simulink model "lab6b"  (R2013b)
settings: Solver=ode3  StartTime=0.0  StopTime=10  FixedStep=0.002  RelTol=1e-3
undefined symbols (not defined in the file or in its folder): HIL
libraries: quarc_library x3
settings Model: SimulationMode=external  ExtModeTrigDuration=1000000  Creator=ee128-aat  LastModifiedBy=ee128-aat
settings SolverCC: PositivePriorityOrder=on
settings DataIOCC: LimitDataPoints=off
settings RTWCC: SystemTargetFile=quarc_win64.tlc  TemplateMakefile=quarc_default_tmf  Description=QUARC Win64 Target  ProcessScript=quarc_win64_make_rtw_hook
settings STFCustomTargetCC: TargetPreCompLibLocation=C:\PROGRA~3\QUARC\lib\2013b\win64\release  GeneratePreprocessorConditionals=Disable all  CombineOutputUpdateFcns=on  GRTInterface=off  SystemTargetFile=quarc_win64.tlc
settings GRTTargetCC: TargetPreCompLibLocation=C:\PROGRA~3\QUARC\lib\2013b\win64\release  ParMdlRefBuildCompliant=off  CompOptLevelCompliant=off  ConcurrentExecutionCompliant=off  MatFileLogging=off  ExtMode=on  ExtModeMexFile=quarc_comm

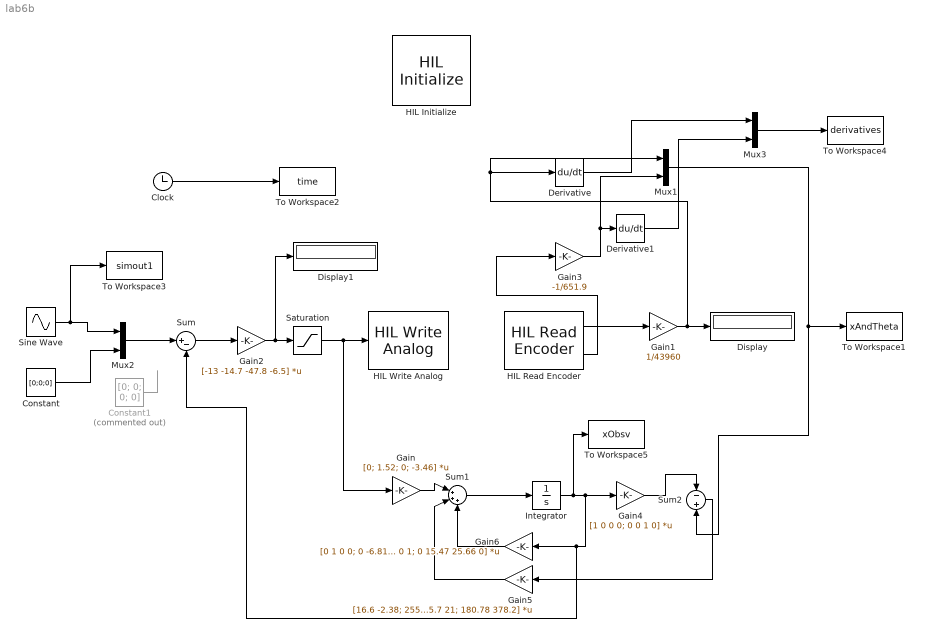
== system lab6b ==
  Clock : Clock
  Constant : Constant  Value=[0;0;0]
  Constant1 : Constant  Commented=on  Value=[0; 0; 0; 0]
  Derivative : Derivative
  Derivative1 : Derivative
  Display : Display
  Display1 : Display
  Gain : Gain  Gain=[0; 1.52; 0; -3.46]  Multiplication=Matrix(K*u)
  Gain1 : Gain  Gain=1/43960
  Gain2 : Gain  Gain=[-13 -14.7 -47.8 -6.5]  Multiplication=Matrix(K*u)
  Gain3 : Gain  Gain=-1/651.9
  Gain4 : Gain  Gain=[1 0 0 0; 0 0 1 0]  Multiplication=Matrix(K*u)
  Gain5 : Gain  Gain=[16.6 -2.38; 255 -5.49; 15.7 21; 180.78 378.2]  Multiplication=Matrix(K*u)
  Gain6 : Gain  Gain=[0 1 0 0; 0 -6.81 -1.5 0; 0 0 0 1; 0 15.47 25.66 0]  Multiplication=Matrix(K*u)
  HIL Initialize : quarc_library/Data Acquisition/Generic/Configuration/HIL Initialize  Priority=-99  object_name=HIL-1  board_type=q2_usb  board_number=0  board_options=d0=digital;d1=digital;led=auto;update_rate=normal;decimation=1  exclusive=off  active=off  hardware_clocks=[0]  clock_modes=[]  initial_clock_frequencies=[]  set_clock_params_at_start=off  set_clock_params_at_switch_in=off  set_clock_frequencies_at_start=off  set_clock_frequencies_at_switch_in=off  analog_input_channels=[0:1]  analog_input_maximums=10  analog_input_minimums=-10  set_analog_input_params_at_start=on  set_analog_input_params_at_switch_in=off  analog_output_channels=[0:1]  analog_output_maximums=10  analog_output_minimums=-10  initial_analog_outputs=[0]  final_analog_outputs=[0]  watchdog_analog_outputs=0  set_analog_output_params_at_start=on  set_analog_output_params_at_switch_in=off  set_analog_outputs_at_start=on  set_analog_outputs_at_switch_in=off  set_analog_outputs_at_terminate=on  set_analog_outputs_at_switch_out=off  set_analog_outputs_on_watchdog=off  digital_input_channels=[]  digital_output_channels=[]  digital_output_configuration=[]  initial_digital_outputs=[1]  final_digital_outputs=[1]  watchdog_digital_outputs=[1]  set_digital_output_params_at_start=off  set_digital_output_params_at_switch_in=off  set_digital_outputs_at_start=on  set_digital_outputs_at_switch_in=off  set_digital_outputs_at_terminate=on  set_digital_outputs_at_switch_out=off  set_digital_outputs_on_watchdog=off  encoder_channels=[0:1]  quadrature=[4]  encoder_filter_frequency=[]  initial_encoder_counts=[0]  set_encoder_params_at_start=on  set_encoder_params_at_switch_in=off  set_encoder_counts_at_start=on  set_encoder_counts_at_switch_in=off  pwm_channels=[]  pwm_modes=[0]  pwm_frequency=1/0.020  pwm_configuration=[]  pwm_alignment=[]  pwm_polarity=[]  pwm_leading_deadband=[]  pwm_trailing_deadband=[]  initial_pwm_outputs=[0]  final_pwm_outputs=[0]  watchdog_pwm_outputs=[0]  set_pwm_params_at_start=on  set_pwm_params_at_switch_in=off  set_pwm_outputs_at_start=on  set_pwm_outputs_at_switch_in=off  set_pwm_outputs_at_terminate=on  set_pwm_outputs_at_switch_out=off  set_pwm_outputs_on_watchdog=off  other_output_channels=[]  initial_other_outputs=[]  final_other_outputs=[]  watchdog_other_outputs=[]  set_other_outputs_at_start=off  set_other_outputs_at_switch_in=off  set_other_outputs_at_terminate=off  set_other_outputs_at_switch_out=off  set_other_outputs_on_watchdog=off
  HIL Read Encoder : quarc_library/Data Acquisition/Generic/Immediate I//O/HIL Read Encoder  object_name=HIL-1  channels=[0:1]  sample_time=qc_get_step_size  active=on  vector_output=off  data_type_mode=Inherit via back propagation  data_type=double
  HIL Write Analog : quarc_library/Data Acquisition/Generic/Immediate I//O/HIL Write Analog  object_name=HIL-1  channels=0  sample_time=-1  active=off  vector_input=off
  Integrator : Integrator
  Mux1 : Mux  Inputs=2
  Mux2 : Mux  Inputs=2
  Mux3 : Mux  Inputs=2
  Saturation : Saturate  UpperLimit=6  LowerLimit=-6
  Sine Wave : Sin  Amplitude=0.05  SampleTime=0
  Sum : Sum  Inputs=|+-
  Sum1 : Sum  Inputs=|+++
  Sum2 : Sum  Inputs=-+
  To Workspace1 : ToWorkspace  VariableName=xAndTheta  SampleTime=-1
  To Workspace2 : ToWorkspace  VariableName=time  SampleTime=-1
  To Workspace3 : ToWorkspace  VariableName=simout1  SampleTime=-1
  To Workspace4 : ToWorkspace  VariableName=derivatives  SampleTime=-1
  To Workspace5 : ToWorkspace  VariableName=xObsv  SampleTime=-1
  wires:
  Clock/1 -> To Workspace2/1
  Gain1/1 -> Display/1, Derivative/1, Mux1/1
  Sum/1 -> Gain2/1
  Saturation/1 -> Gain/1, HIL Write Analog/1
  Gain3/1 -> Mux1/2, Derivative1/1
  HIL Read Encoder/1 -> Gain1/1
  Mux1/1 -> To Workspace1/1, Sum2/2
  HIL Read Encoder/2 -> Gain3/1
  Gain2/1 -> Display1/1, Saturation/1
  Sine Wave/1 -> To Workspace3/1, Mux2/1
  Constant/1 -> Mux2/2
  Gain/1 -> Sum1/1
  Sum1/1 -> Integrator/1
  Integrator/1 -> Gain6/1, Sum/2, Gain4/1, To Workspace5/1
  Gain4/1 -> Sum2/1
  Sum2/1 -> Gain5/1
  Gain5/1 -> Sum1/2
  Gain6/1 -> Sum1/3
  Constant1/1 -> ?
  Derivative/1 -> Mux3/1
  Derivative1/1 -> Mux3/2
  Mux3/1 -> To Workspace4/1
  Mux2/1 -> Sum/1
